simulink model "mElegooSonarControlAndroid"  (R2022b)
settings: Solver=FixedStepDiscrete  StartTime=0.0  StopTime=10.0  FixedStep=0.1  RelTol=1e-3
libraries: androidcommunicationlib x2, androiduilib x1
settings Model: Creator=The MathWorks, Inc.  LastModifiedBy=ivang
settings SolverCC: AlgebraicLoopSolver=TrustRegion
settings OptimizationCC: EnhancedBackFolding=on  PassReuseOutputArgsThreshold=0  MaxStackSize=64  OptimizeBlockOrder=speed  DifferentSizesBufferReuse=on  OptimizationCustomize=off
settings DebuggingCC: ParameterTunabilityLossMsg=error  UnconnectedInputMsg=warning  UnconnectedOutputMsg=warning  UnconnectedLineMsg=warning  SymbolicDimsDataTypeCodeGenerationDiagnostic=none  SFMachineParentedDataDiag=warning
settings HardwareCC: ProdBitPerPointer=32  ProdBitPerSizeT=32  ProdBitPerPtrDiffT=32  ProdLargestAtomicInteger=Long  ProdLargestAtomicFloat=Double  ProdWordSize=32  ProdHWDeviceType=ARM Compatible->ARM Cortex  UseEmbeddedCoderFeatures=off  UseSimulinkCoderFeatures=off
settings ModelReferenceCC: EnableRefExpFcnMdlSchedulingChecks=on
settings SFSimCC: MATLABDynamicMemAlloc=off
settings RTWCC: Description=Embedded Coder  SystemTargetFile=ert.tlc  HardwareBoard=Android Device  TLCOptions="-aInlineSetEventsForThisBaseRateFcn=TLC_FALSE -aSuppressMultiTaskScheduler=TLC_FALSE  -aRateBasedStepFcn=0"  TemplateMakefile=ert_default_tmf  GenerateReport=on  RTWVerbose=off  Toolchain=Android SDK/NDK Tools  LaunchReport=on
settings CodeAppCC: ForceParamTrailComments=on  OperatorAnnotations=on
settings ERTTargetCC: ERTCustomFileBanners=off  SupportContinuousTime=on  SupportNonInlinedSFcns=on  RemoveResetFunc=off  ModelStepFunctionPrototypeControlCompliant=off

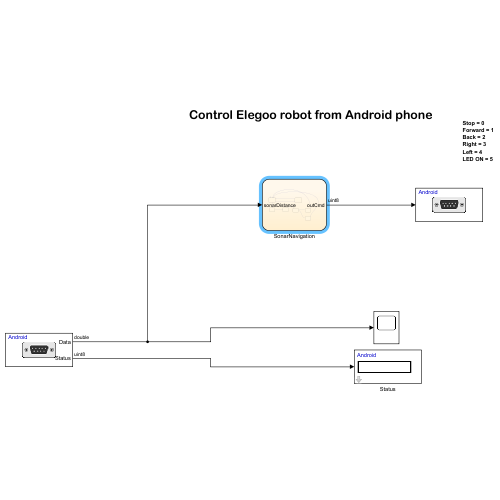
[thumbnail: Simulink's stored preview of the top-level diagram]
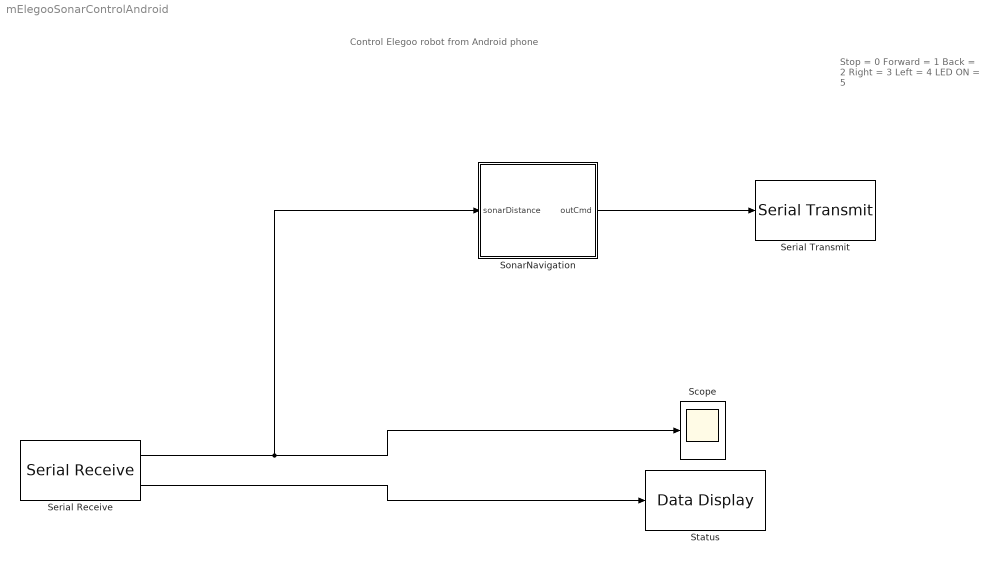
== system mElegooSonarControlAndroid ==
  note: Control Elegoo robot from Android phone
  note: Stop = 0
      | Forward = 1
      | Back = 2
      | Right = 3
      | Left = 4
      | LED ON = 5
  Scope : Scope
  Serial Receive : androidcommunicationlib/Serial Receive  DataType=uint8  DataSize=1  SampleTime=0.1
  Serial Transmit : androidcommunicationlib/Serial Transmit
  SonarNavigation : Stateflow chart  TreatAsAtomicUnit=on
  Status : androiduilib/Data Display  DataDisplayId=mElegooSonarControlAndroid/Status  Format=Integer  Precision=6  SimulateUsing=Code generation  blockPlatform=Android
  wires:
  Serial Receive/2 -> Status/1
  SonarNavigation/1(outCmd) -> Serial Transmit/1
  Serial Receive/1 -> Scope/1, SonarNavigation/1(sonarDistance)

== stateflow chart mElegooSonarControlAndroid/SonarNavigation ==
  state Entry
    outCmd = 0;
  state MoveForward
    outCmd = 1;
  state MoveBack1
    outCmd = 2;
  state MoveBack2
    outCmd = 0;
  state MoveBack3
    outCmd = 0;
  state MoveRight
    outCmd = 3;
  state MoveLeft
    outCmd = 4;
  MoveRight -> Entry : [after(500, msec)]
  MoveLeft -> Entry : [after(500, msec)]
  (default) -> Entry
  MoveForward -> Entry : [after(500, msec)]
  Entry -> MoveForward [order 1] : [after(500, msec)]
  Entry -> MoveBack1 [order 2] : [sonarDistance < 10]
  MoveBack2 -> MoveBack3 : [after(500, msec)]
  MoveBack1 -> MoveBack2 : [after(100, msec)]
  MoveBack3 -> MoveRight [order 1] : [randi([1, 10]) > 5]
  MoveBack3 -> MoveLeft [order 2]
  data: outCmd output uint8 =uint8(0); sonarDistance input uint8
